simulink model "Simulation_DOA_rearanged"  (R2020b)
settings: Solver=ode4  StartTime=0.0  StopTime=timeToStop  FixedStep=1e-7  RelTol=1e-3
values from neighbouring files (symbols this model uses):
  f_range = [20e3 45e3]    [Init.m]
  FFT_LENGTH = 256    [Init.m]
  noise_on_off = false    [Init.m]
  noise_type = 1    [Init.m]
  Sampling_rate = 256e3    (= 256000)    [Init.m]
  timePerSample = 1/250e3    (= 4e-06)    [Init.m]
undefined symbols (not defined in the file or in its folder): Coeff_rect, InvMp, ProjectRate, RotX, runSim, SampleEstimate
libraries: dspsigops x25, dspsrcs4 x8, dsphdlmathfun x4, dsphdlxfrm x4, simulink x1, hdlsllib x1
(part 1 of 2)
settings Model: Creator=tigro  LastModifiedBy=franc
settings OptimizationCC: BlockReduction=off  ConditionallyExecuteInputs=off  DefaultParameterBehavior=Inlined  OptimizeBlockIOStorage=off  EnhancedBackFolding=on  PassReuseOutputArgsAs=Individual arguments  OptimizeBlockOrder=speed  DifferentSizesBufferReuse=on  EfficientTunableParamExpr=on
settings DebuggingCC: AlgebraicLoopMsg=error  ParameterOverflowMsg=none  ParameterTunabilityLossMsg=error
settings HardwareCC: ProdBitPerPointer=32  ProdBitPerSizeT=32  ProdBitPerPtrDiffT=32  ProdLargestAtomicFloat=None  ProdIntDivRoundTo=Undefined  ProdEndianess=Unspecified  ProdWordSize=32  ProdHWDeviceType=ASIC/FPGA->ASIC/FPGA  TargetBitPerPointer=64  TargetBitPerSizeT=64  TargetBitPerPtrDiffT=64  TargetLongLongMode=on  TargetIntDivRoundTo=Zero  TargetEndianess=LittleEndian  TargetWordSize=64  TargetHWDeviceType=Generic->Custom  ProdEqTarget=off
settings SFSimCC: MATLABDynamicMemAlloc=off
settings RTWCC: Description=SystemVerilog DPI Component Generator  SystemTargetFile=systemverilog_dpi_ert.tlc  TemplateMakefile=systemverilog_dpi_ert_default_tmf
settings CodeAppCC: ForceParamTrailComments=on  IgnoreCustomStorageClasses=off  MaxIdLength=256  OperatorAnnotations=on  SimulinkDataObjDesc=on  SFDataObjDesc=on  InsertBlockDesc=on
settings DPIERTTargetCC: TargetFcnLib=ansi_tfl_table_tmw.mat  GenFloatMathFcnCalls=NOT IN USE  TargetLangStandard=C89/C90 (ANSI)  CodeReplacementLibrary=None  UtilityFuncGeneration=Auto  MultiwordTypeDef=System defined  MultiwordLength=2048  DynamicStringBufferSize=256  GenerateFullHeader=on  InferredTypesCompatibility=off  GenerateSampleERTMain=off  GenerateTestInterfaces=off  ModelReferenceCompliant=on  ParMdlRefBuildCompliant=on  CompOptLevelCompliant=off  ConcurrentExecutionCompliant=off  IncludeMdlTerminateFcn=on  CombineOutputUpdateFcns=off  CombineSignalStateStructs=on  GroupInternalDataByFunction=off  SuppressErrorStatus=off  IncludeFileDelimiter=Auto  ERTCustomFileBanners=on  SupportAbsoluteTime=on  LogVarNameModifier=rt_  MatFileLogging=off  CodeInterfacePackaging=Reusable function  PurelyIntegerCode=off  SupportNonFinite=on  SupportComplex=on  SupportContinuousTime=on  SupportNonInlinedSFcns=on  RemoveDisableFunc=off  RemoveResetFunc=on  SupportVariableSizeSignals=off  ParenthesesLevel=Nominal  CastingMode=Nominal  MATLABClassNameForMDSCustomization=Simulink.SoftwareTarget.TargetSpecificTriggerConfigurationBase  ModelStepFunctionPrototypeControlCompliant=on  CPPClassGenCompliant=off  AutosarCompliant=off  MDXCompliant=off  GRTInterface=off  GenerateAllocFcn=on  UseToolchainInfoCompliant=on  GenerateSharedConstants=on  CoderGroups=[]  AccessMethods=[]  LookupTableObjectStructAxisOrder=1,2,3,4,...  LUTObjectStructOrderExplicitValues=Size,Breakpoints,Table  LUTObjectStructOrderEvenSpacing=Size,Breakpoints,Table  ArrayLayout=Column-major  UnsupportedSFcnMsg=error  ERTHeaderFileRootName=$R$E  ERTSourceFileRootName=$R$E  ERTDataFileRootName=$R_data  GenerateASAP2=off  DSAsUniqueAccess=off  ExtMode=off  ExtModeTransport=0  ExtModeStaticAlloc=off  ExtModeStaticAllocSize=1000000  ExtModeTesting=off  ExtModeMexFile=ext_comm  ExtModeIntrfLevel=Level1  InlinedParameterPlacement=NonHierarchical  TargetOS=BareBoardExample  MultiInstanceErrorCode=Error  RootIOFormat=Part of model data structure  RTWCAPISignals=on  RTWCAPIParams=off  RTWCAPIStates=off  RTWCAPIRootIO=off  ERTSrcFileBannerTemplate=ert_code_template.cgt  ERTHdrFileBannerTemplate=ert_code_template.cgt  ERTDataSrcFileTemplate=ert_code_template.cgt  ERTDataHdrFileTemplate=ert_code_template.cgt  ERTCustomFileTemplate=example_file_process.tlc  EnableDataOwnership=off  SignalDisplayLevel=10  ParamTuneLevel=10  GlobalDataDefinition=Auto  DataDefinitionFile=global.c  GlobalDataReference=Auto  ERTFilePackagingFormat=Modular  RateTransitionBlockCode=Inline  DataReferenceFile=global.h  PreserveExpressionOrder=off  PreserveIfCondition=off  ConvertIfToSwitch=on  PreserveExternInFcnDecls=on  PreserveStaticInFcnDecls=on  SuppressUnreachableDefaultCases=on  EnableSignedLeftShifts=on  EnableSignedRightShifts=on  IndentStyle=K&R  IndentSize=2  NewlineStyle=Default  MaxLineWidth=80  EnableUserReplacementTypes=off  MaxIdInt64=MAX_int64_T  MinIdInt64=MIN_int64_T  MaxIdUint64=MAX_uint64_T  MaxIdInt32=MAX_int32_T  MinIdInt32=MIN_int32_T  MaxIdUint32=MAX_uint32_T  MaxIdInt16=MAX_int16_T  MinIdInt16=MIN_int16_T  MaxIdUint16=MAX_uint16_T  MaxIdInt8=MAX_int8_T  MinIdInt8=MIN_int8_T  MaxIdUint8=MAX_uint8_T  BooleanTrueId=true  BooleanFalseId=false  MemSecPackage=--- None ---  MemSecDataConstants=Default  MemSecDataIO=Default  MemSecDataInternal=Default  MemSecDataParameters=Default  MemSecFuncInitTerm=Default  MemSecFuncExecute=Default  MemSecFuncSharedUtil=Default  GroupConstants=Default  GroupRootInputs=Default  GroupRootOutputs=Default  GroupInternal=Default  GroupParameters=Default  GroupDataTransfer=Default  GroupSharedLocalDataStores=Default  GroupInstanceSpecificParameters=Default  GroupModelData=Default  ArrayContainerType=C-style array  DPICustomizeSystemVerilogCode=off  DPISystemVerilogTemplate=svdpi_event.vgt  DPIReportRunTimeError=off  DPIRunTimeErrorSeverity=Fatal  DPIGenerateTestBench=off  DPITestBenchSimulator=Mentor Graphics Questasim  DPITestPointAccessFcnInterface=None  DPIFixedPointDataType=CompatibleCType  DPIPortConnection=Port list  DPICompositeDataType=Flattened

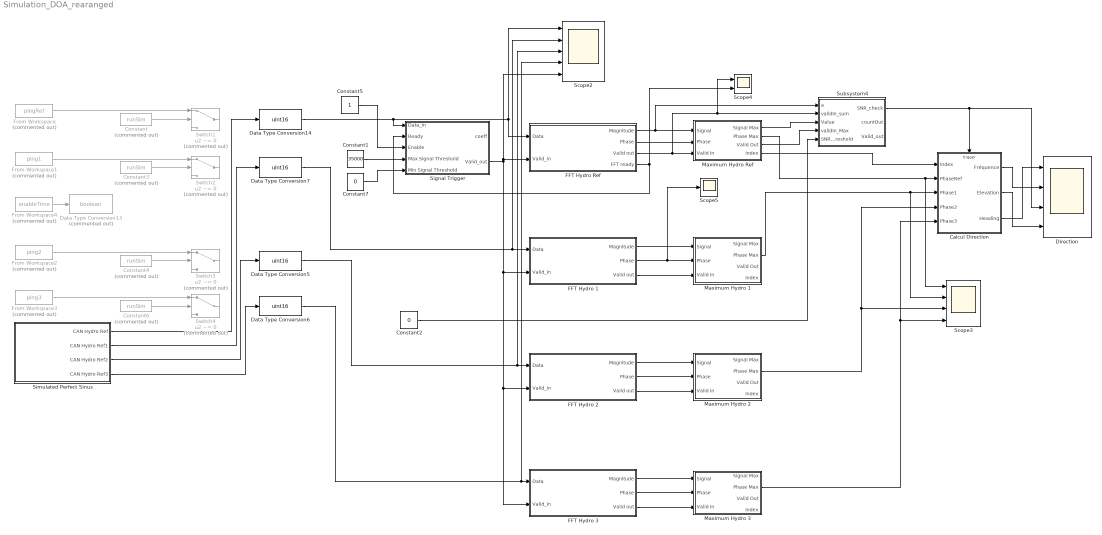
== system Simulation_DOA_rearanged ==
  Calcul Direction : Subsystem
  Constant{,3..4,6} (4 alike) : Constant  Commented=on  Value=runSim  SampleTime=-1
  Constant1 : Constant  Value=35000  OutDataTypeStr=uint16  SampleTime=-1
  Constant2 : Constant  Value=0  OutDataTypeStr=uint16  SampleTime=-1
  Constant5 : Constant  OutDataTypeStr=boolean
  Constant7 : Constant  Value=0  OutDataTypeStr=uint16  SampleTime=-1
  Data Type Conversion13 : DataTypeConversion  Commented=on  OutDataTypeStr=boolean
  Data Type Conversion{5..7,14} (4 alike) : DataTypeConversion  OutMax=[65535]  OutDataTypeStr=uint16
  Direction : Scope  NumInputPorts=4
  FFT Hydro 1 : Subsystem
  FFT Hydro 2 : Subsystem
  FFT Hydro 3 : Subsystem
  FFT Hydro Ref : Subsystem
  From Workspace : FromWorkspace  Commented=on  VariableName=pingRef  SampleTime=1/SampleEstimate  Interpolate=off  OutputAfterFinalValue=Setting to zero
  From Workspace1 : FromWorkspace  Commented=on  VariableName=ping1  SampleTime=1/SampleEstimate  Interpolate=off  OutputAfterFinalValue=Setting to zero
  From Workspace2 : FromWorkspace  Commented=on  VariableName=ping2  SampleTime=1/SampleEstimate  Interpolate=off  OutputAfterFinalValue=Setting to zero
  From Workspace3 : FromWorkspace  Commented=on  VariableName=ping3  SampleTime=1/SampleEstimate  Interpolate=off  OutputAfterFinalValue=Setting to zero
  From Workspace4 : FromWorkspace  Commented=on  VariableName=enableTime  SampleTime=1/ProjectRate  Interpolate=off  OutputAfterFinalValue=Setting to zero
  Maximum Hydro 1 : Subsystem
  Maximum Hydro 2 : Subsystem
  Maximum Hydro 3 : Subsystem
  Maximum Hydro Ref : Subsystem
  Scope2 : Scope  NumInputPorts=5
  Scope3 : Scope  NumInputPorts=4
  Scope4 : Scope  NumInputPorts=2
  Scope5 : Scope
  Signal Trigger : Subsystem
  Simulated Perfect Sinus : Subsystem
  Subsystem4 : Subsystem
  Switch{1..4} (4 alike) : Switch  Commented=on  Criteria=u2 ~= 0
  wires:
  Maximum Hydro Ref/1(Signal Max) -> Subsystem4/3(" Value")
  Data Type Conversion14/1 -> Signal Trigger/1(Data_in), Scope2/1, FFT Hydro Ref/1(Data)
  Data Type Conversion7/1 -> Scope2/2, FFT Hydro 1/1(Data)
  Data Type Conversion6/1 -> FFT Hydro 3/1(Data), Scope2/4
  FFT Hydro Ref/2(Phase) -> Maximum Hydro Ref/2(Phase)
  Maximum Hydro Ref/2(Phase Max) -> Scope3/1, Calcul Direction/2(PhaseRef)
  Maximum Hydro 1/2(Phase Max) -> Scope3/2, Calcul Direction/3(Phase1)
  Maximum Hydro 2/2(Phase Max) -> Calcul Direction/4(Phase2), Scope3/3
  Maximum Hydro 3/2(Phase Max) -> Calcul Direction/5(Phase3), Scope3/4
  Signal Trigger/2(Valid_out) -> Scope2/5, FFT Hydro Ref/2(Valid_in), FFT Hydro 3/2(Valid_in), FFT Hydro 2/2(Valid_in), FFT Hydro 1/2(Valid_in)
  FFT Hydro 1/1(Magnitude) -> Maximum Hydro 1/1(Signal)
  FFT Hydro 1/2(Phase) -> Scope5/1, Maximum Hydro 1/2(Phase)
  FFT Hydro 1/3(Valid out) -> Maximum Hydro 1/3(Valid In)
  FFT Hydro 2/1(Magnitude) -> Maximum Hydro 2/1(Signal)
  FFT Hydro 2/2(Phase) -> Maximum Hydro 2/2(Phase)
  FFT Hydro 2/3(Valid out) -> Maximum Hydro 2/3(Valid In)
  FFT Hydro 3/1(Magnitude) -> Maximum Hydro 3/1(Signal)
  FFT Hydro 3/2(Phase) -> Maximum Hydro 3/2(Phase)
  FFT Hydro 3/3(Valid out) -> Maximum Hydro 3/3(Valid In)
  Maximum Hydro Ref/3(Valid Out) -> Subsystem4/4(validIn_Max)
  FFT Hydro Ref/3(Valid out) -> Maximum Hydro Ref/3(Valid In), Scope4/1, Subsystem4/2(validIn_sum)
  Calcul Direction/1(Fréquence) -> Direction/2
  FFT Hydro Ref/1(Magnitude) -> Maximum Hydro Ref/1(Signal), Subsystem4/1(a)
  Subsystem4/1(SNR_check) -> Calcul Direction/Trigger, Direction/3
  Constant1/1 -> Signal Trigger/4(Max Signal Threshold)
  Constant2/1 -> Subsystem4/5(SNR_Threshold)
  Calcul Direction/2(Elevation) -> Direction/4
  From Workspace/1 -> Switch1/1
  From Workspace1/1 -> Switch2/1
  From Workspace2/1 -> Switch3/1
  From Workspace3/1 -> Switch4/1
  Constant/1 -> Switch1/2
  Constant3/1 -> Switch2/2
  Constant4/1 -> Switch3/2
  Constant6/1 -> Switch4/2
  FFT Hydro Ref/4(FFT ready) -> Scope4/2, Signal Trigger/2(Ready)
  From Workspace4/1 -> Data Type Conversion13/1
  Simulated Perfect Sinus/1(CAN Hydro Ref) -> Data Type Conversion14/1
  Simulated Perfect Sinus/2(CAN Hydro Ref1) -> Data Type Conversion7/1
  Simulated Perfect Sinus/3(CAN Hydro Ref2) -> Data Type Conversion5/1
  Simulated Perfect Sinus/4(CAN Hydro Ref3) -> Data Type Conversion6/1
  Constant7/1 -> Signal Trigger/5(Min Signal Threshold)
  Data Type Conversion5/1 -> Scope2/3, FFT Hydro 2/1(Data)
  Maximum Hydro Ref/4(Index) -> Calcul Direction/1(Index)
  Calcul Direction/3(Heading) -> Direction/1
  Constant5/1 -> Signal Trigger/3(Enable)

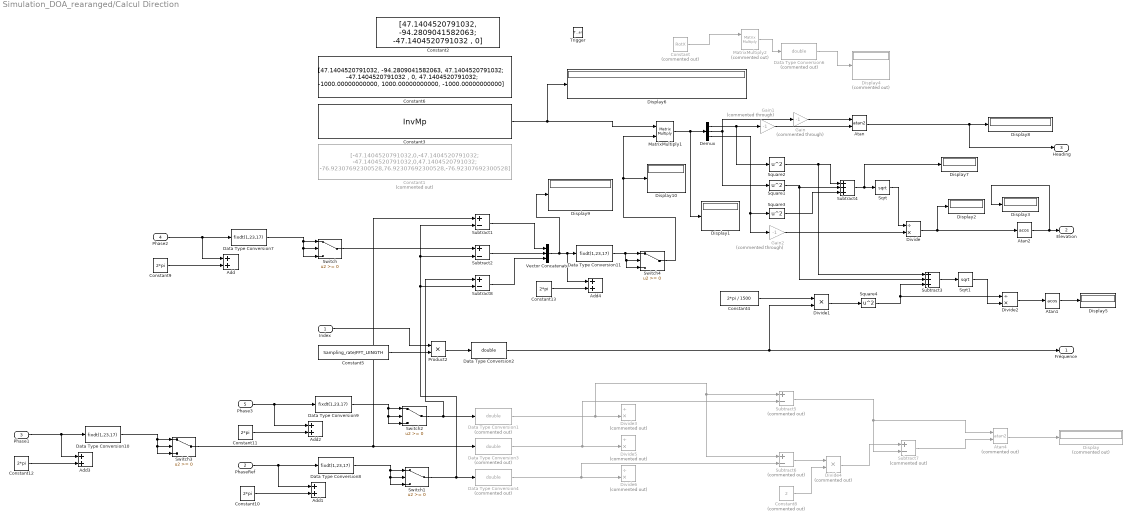
== system Simulation_DOA_rearanged/Calcul Direction ==
  Index : Inport
  PhaseRef : Inport  Port=2
  Phase1 : Inport  Port=3
  Phase2 : Inport  Port=4
  Phase3 : Inport  Port=5
  Trigger : TriggerPort  VariantControl=Variant  PortDimensions=1
  Add{,1..4} (5 alike) : Sum
  Atan : Trigonometry  Operator=atan2  ApproximationMethod=CORDIC  OutputSignalType=real
  Atan1 : Trigonometry  Operator=acos  ApproximationMethod=CORDIC  OutputSignalType=real
  Atan2 : Trigonometry  Operator=acos  ApproximationMethod=CORDIC  OutputSignalType=real
  Atan4 : Trigonometry  Commented=on  Operator=atan2  ApproximationMethod=CORDIC  OutputSignalType=real
  Constant : Constant  Commented=on  Value=RotX
  Constant1 : Constant  Commented=on  Value=|  VectorParams1D=off  OutDataTypeStr=fixdt(1,15,7)
      | [-47.1404520791032,0,-47.1404520791032; -47.1404520791032,0,47.1404520791032;
      | -76.92307692300528,76.92307692300528,-76.92307692300528]
  Constant{9..13} (5 alike) : Constant  Value=2*pi  OutDataTypeStr=fixdt(0,16,12)  SampleTime=-1
  Constant2 : Constant  Value=|  VectorParams1D=off  OutDataTypeStr=fixdt(1,15,7)
      | [47.1404520791032,    -94.2809041582063;
      | -47.1404520791032 ,   0]
  Constant3 : Constant  Value=InvMp  VectorParams1D=off  OutDataTypeStr=fixdt(1,32,16)
  Constant4 : Constant  Value=2*pi / 1500
  Constant5 : Constant  Value=Sampling_rate/FFT_LENGTH  OutDataTypeStr=Inherit: Inherit via back propagation  SampleTime=-1
  Constant6 : Constant  Value=|  VectorParams1D=off  OutDataTypeStr=fixdt(1,15,7)
      | [47.1404520791032,    -94.2809041582063,    47.1404520791032;
      | -47.1404520791032 ,   0,    47.1404520791032;
      | -1000.00000000000,   1000.00000000000,    -1000.00000000000]
  Constant8 : Constant  Commented=on  Value=2  OutDataTypeStr=uint8
  Data Type Conversion{1,3..4,6} (4 alike) : DataTypeConversion  Commented=on  OutDataTypeStr=double
  Data Type Conversion{7..11} (5 alike) : DataTypeConversion  OutDataTypeStr=fixdt(1,23,17)
  Data Type Conversion2 : DataTypeConversion  OutDataTypeStr=double
  Demux : Demux  Outputs=3
  Display : Display  Commented=on
      settings: Decimation=8
  Display{1..3,5..10} (9 alike) : Display
      Display8 settings: Decimation=8
  Display4 : Display  Commented=on
  Divide : Product  Inputs=/*
  Divide1 : Product  Inputs=**  RndMeth=Zero  SaturateOnIntegerOverflow=on
  Divide2 : Product  Inputs=/*
  Divide3 : Product  Commented=on  Inputs=/*  RndMeth=Zero  SaturateOnIntegerOverflow=on
  Divide4 : Product  Commented=on  Inputs=**  RndMeth=Zero  SaturateOnIntegerOverflow=on
  Divide5 : Product  Commented=on  Inputs=/*  RndMeth=Zero  SaturateOnIntegerOverflow=on
  Divide6 : Product  Commented=on  Inputs=/*  RndMeth=Zero  SaturateOnIntegerOverflow=on
  Gain : Gain  Commented=through  Gain=-1
  Gain1 : Gain  Commented=through  Gain=-1
  Gain2 : Gain  Commented=through  Gain=-1
  MatrixMultiply1 : Product  Multiplication=Matrix(*)
  MatrixMultiply2 : Product  Commented=on  Multiplication=Matrix(*)
  Product2 : Product
  Sqrt : Sqrt  OutDataTypeStr=double  SaturateOnIntegerOverflow=on
  Sqrt1 : Sqrt  OutDataTypeStr=double  SaturateOnIntegerOverflow=on
  Square{1..4} (4 alike) : Math  Operator=square  SignedPower=on  RndMeth=Zero  SaturateOnIntegerOverflow=on  OutDataTypeStr=Inherit: Inherit via internal rule
  Subtract1 : Sum  Inputs=+-
  Subtract2 : Sum  Inputs=+-
  Subtract3 : Sum  Inputs=+++
  Subtract4 : Sum  Inputs=+++
  Subtract5 : Sum  Commented=on  Inputs=+-
  Subtract6 : Sum  Commented=on  Inputs=+-
  Subtract7 : Sum  Commented=on  Inputs=+-
  Subtract8 : Sum  Inputs=+-
  Switch{,1..4} (5 alike) : Switch
  Vector Concatenate : Concatenate  NumInputs=3  Mode=Multidimensional array
  Fréquence : Outport  InitialOutput=0
  Elevation : Outport  Port=2  InitialOutput=0
  Heading : Outport  Port=3  InitialOutput=0
  wires:
  Constant5/1 -> Product2/2
  Square2/1 -> Subtract3/1, Subtract4/1
  Demux/1 -> Square2/1, Gain1/1
  Product2/1 -> Data Type Conversion2/1
  Subtract4/1 -> Display7/1, Sqrt/1
  Index/1 -> Product2/1
  Square1/1 -> Subtract3/2, Subtract4/2
  Square3/1 -> Subtract4/3
  Sqrt/1 -> Divide/1
  Atan2/1 -> Display3/1, Elevation/1
  Demux/2 -> Gain/1, Square1/1
  MatrixMultiply1/1 -> Display1/1, Demux/1
  Demux/3 -> Gain2/1, Square3/1
  Constant3/1 -> Display6/1, MatrixMultiply1/1
  Constant/1 -> MatrixMultiply2/1
  MatrixMultiply2/1 -> Data Type Conversion6/1
  Data Type Conversion6/1 -> Display4/1
  Constant4/1 -> Divide1/1
  Divide1/1 -> Square4/1
  Subtract3/1 -> Sqrt1/1
  Square4/1 -> Divide2/1, Subtract3/3
  Sqrt1/1 -> Divide2/2
  Divide2/1 -> Atan1/1
  Atan1/1 -> Display5/1
  Vector Concatenate/1 -> Display9/1, Add4/1, Data Type Conversion11/1
  Divide4/1 -> Subtract7/1
  Subtract7/1 -> Atan4/2
  Subtract6/1 -> Divide4/1
  Constant8/1 -> Divide4/2
  Subtract5/1 -> Atan4/1, Subtract7/2
  Atan4/1 -> Display/1
  Data Type Conversion1/1 -> Divide3/2, Subtract6/1, Subtract5/1
  Data Type Conversion3/1 -> Divide5/2, Subtract5/2
  Data Type Conversion4/1 -> Divide6/2, Subtract6/2
  Data Type Conversion2/1 -> Divide1/2, Fréquence/1
  Atan/1 -> Heading/1, Display8/1
  Switch/1 -> Subtract2/1
  Constant9/1 -> Add/2
  Phase2/1 -> Add/1, Data Type Conversion7/1
  Data Type Conversion7/1 -> Switch/3, Switch/2, Switch/1
  Constant10/1 -> Add1/2
  Data Type Conversion8/1 -> Switch1/3, Switch1/2, Switch1/1
  Constant11/1 -> Add2/2
  Data Type Conversion9/1 -> Switch2/3, Switch2/2, Switch2/1
  Constant12/1 -> Add3/2
  Data Type Conversion10/1 -> Switch3/3, Switch3/2, Switch3/1
  Switch1/1 -> Subtract8/2, Subtract2/2, Subtract1/2, Data Type Conversion4/1
  PhaseRef/1 -> Add1/1, Data Type Conversion8/1
  Switch2/1 -> Subtract8/1, Data Type Conversion1/1
  Phase3/1 -> Add2/1, Data Type Conversion9/1
  Switch3/1 -> Data Type Conversion3/1, Subtract1/1
  Phase1/1 -> Add3/1, Data Type Conversion10/1
  Data Type Conversion11/1 -> Switch4/3, Switch4/2, Switch4/1
  Constant13/1 -> Add4/2
  Switch4/1 -> Display10/1, MatrixMultiply1/2
  Subtract1/1 -> Vector Concatenate/1
  Subtract2/1 -> Vector Concatenate/2
  Subtract8/1 -> Vector Concatenate/3
  Gain/1 -> Atan/1
  Gain1/1 -> Atan/2
  Divide/1 -> Atan2/1, Display2/1
  Gain2/1 -> Divide/2

== system Simulation_DOA_rearanged/FFT Hydro 1 ==
  Data : Inport
  Valid_in : Inport  Port=2
  Complex to Magnitude-Angle HDL Optimized : dsphdlmathfun/Complex to Magnitude-Angle HDL Optimized  NumIterationsSource=Property  NumIterations=CORDIC_Estimation  OutputFormat=Magnitude and angle  AngleFormat=Radians  ScaleOutput=on  SimulateUsing=Code generation
      settings: SourceProductBaseCode=DS
  FFT HDL Optimized : dsphdlxfrm/FFT HDL Optimized  FFTLength=FFT_LENGTH  Architecture=Burst Radix 2  ComplexMultiplication=Use 3 multipliers and 5 adders  BitReversedOutput=off  BitReversedInput=off  Normalize=on  SimulateUsing=Code generation  RoundingMethod=Floor  ResetInputPort=off  StartOutputPort=off  EndOutputPort=on
      settings: SourceProductBaseCode=DS
  Magnitude : Outport
  Phase : Outport  Port=2
  Valid out : Outport  Port=3
  wires:
  Valid_in/1 -> FFT HDL Optimized/2
  FFT HDL Optimized/1 -> Complex to Magnitude-Angle HDL Optimized/1
  Complex to Magnitude-Angle HDL Optimized/1 -> Magnitude/1
  Complex to Magnitude-Angle HDL Optimized/2 -> Phase/1
  Data/1 -> FFT HDL Optimized/1
  FFT HDL Optimized/3 -> Complex to Magnitude-Angle HDL Optimized/2
  Complex to Magnitude-Angle HDL Optimized/3 -> Valid out/1

== system Simulation_DOA_rearanged/FFT Hydro 2 ==
  Data : Inport
  Valid_in : Inport  Port=2
  Complex to Magnitude-Angle HDL Optimized : dsphdlmathfun/Complex to Magnitude-Angle HDL Optimized  NumIterationsSource=Property  NumIterations=CORDIC_Estimation  OutputFormat=Magnitude and angle  AngleFormat=Radians  ScaleOutput=on  SimulateUsing=Code generation
      settings: SourceProductBaseCode=DS
  FFT HDL Optimized : dsphdlxfrm/FFT HDL Optimized  FFTLength=FFT_LENGTH  Architecture=Burst Radix 2  ComplexMultiplication=Use 3 multipliers and 5 adders  BitReversedOutput=off  BitReversedInput=off  Normalize=on  SimulateUsing=Code generation  RoundingMethod=Floor  ResetInputPort=off  StartOutputPort=off  EndOutputPort=on
      settings: SourceProductBaseCode=DS
  Magnitude : Outport
  Phase : Outport  Port=2
  Valid out : Outport  Port=3
  wires:
  Valid_in/1 -> FFT HDL Optimized/2
  FFT HDL Optimized/1 -> Complex to Magnitude-Angle HDL Optimized/1
  Complex to Magnitude-Angle HDL Optimized/1 -> Magnitude/1
  Complex to Magnitude-Angle HDL Optimized/2 -> Phase/1
  Data/1 -> FFT HDL Optimized/1
  FFT HDL Optimized/3 -> Complex to Magnitude-Angle HDL Optimized/2
  Complex to Magnitude-Angle HDL Optimized/3 -> Valid out/1

== system Simulation_DOA_rearanged/FFT Hydro 3 ==
  Data : Inport
  Valid_in : Inport  Port=2
  Complex to Magnitude-Angle HDL Optimized : dsphdlmathfun/Complex to Magnitude-Angle HDL Optimized  NumIterationsSource=Property  NumIterations=CORDIC_Estimation  OutputFormat=Magnitude and angle  AngleFormat=Radians  ScaleOutput=on  SimulateUsing=Code generation
      settings: SourceProductBaseCode=DS
  FFT HDL Optimized : dsphdlxfrm/FFT HDL Optimized  FFTLength=FFT_LENGTH  Architecture=Burst Radix 2  ComplexMultiplication=Use 3 multipliers and 5 adders  BitReversedOutput=off  BitReversedInput=off  Normalize=on  SimulateUsing=Code generation  RoundingMethod=Floor  ResetInputPort=off  StartOutputPort=off  EndOutputPort=on
      settings: SourceProductBaseCode=DS
  Magnitude : Outport
  Phase : Outport  Port=2
  Valid out : Outport  Port=3
  wires:
  Valid_in/1 -> FFT HDL Optimized/2
  FFT HDL Optimized/1 -> Complex to Magnitude-Angle HDL Optimized/1
  Complex to Magnitude-Angle HDL Optimized/1 -> Magnitude/1
  Complex to Magnitude-Angle HDL Optimized/2 -> Phase/1
  Data/1 -> FFT HDL Optimized/1
  FFT HDL Optimized/3 -> Complex to Magnitude-Angle HDL Optimized/2
  Complex to Magnitude-Angle HDL Optimized/3 -> Valid out/1

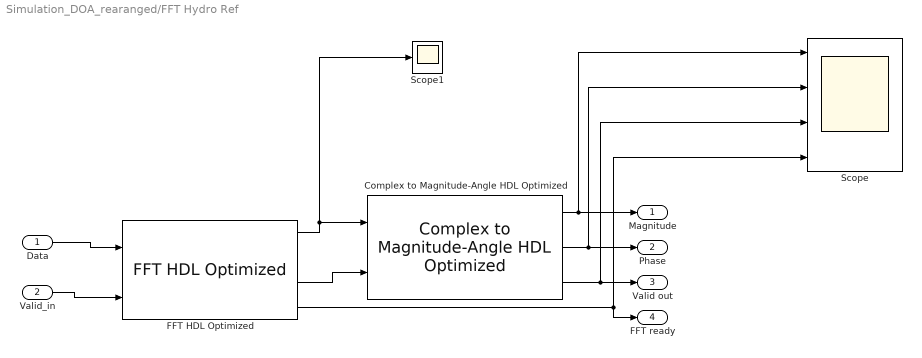
== system Simulation_DOA_rearanged/FFT Hydro Ref ==
  Data : Inport
  Valid_in : Inport  Port=2
  Complex to Magnitude-Angle HDL Optimized : dsphdlmathfun/Complex to Magnitude-Angle HDL Optimized  NumIterationsSource=Property  NumIterations=CORDIC_Estimation  OutputFormat=Magnitude and angle  AngleFormat=Radians  ScaleOutput=on  SimulateUsing=Code generation
      settings: SourceProductBaseCode=DS
  FFT HDL Optimized : dsphdlxfrm/FFT HDL Optimized  FFTLength=FFT_LENGTH  Architecture=Burst Radix 2  ComplexMultiplication=Use 3 multipliers and 5 adders  BitReversedOutput=off  BitReversedInput=off  Normalize=on  SimulateUsing=Code generation  RoundingMethod=Floor  ResetInputPort=off  StartOutputPort=off  EndOutputPort=on
      settings: SourceProductBaseCode=DS
  Scope : Scope  NumInputPorts=4
  Scope1 : Scope
  Magnitude : Outport
  Phase : Outport  Port=2
  Valid out : Outport  Port=3
  FFT ready : Outport  Port=4
  wires:
  Valid_in/1 -> FFT HDL Optimized/2
  FFT HDL Optimized/1 -> Complex to Magnitude-Angle HDL Optimized/1, Scope1/1
  Complex to Magnitude-Angle HDL Optimized/1 -> Scope/1, Magnitude/1
  Complex to Magnitude-Angle HDL Optimized/2 -> Scope/2, Phase/1
  Data/1 -> FFT HDL Optimized/1
  FFT HDL Optimized/3 -> Complex to Magnitude-Angle HDL Optimized/2
  Complex to Magnitude-Angle HDL Optimized/3 -> Scope/3, Valid out/1
  FFT HDL Optimized/4 -> FFT ready/1, Scope/4

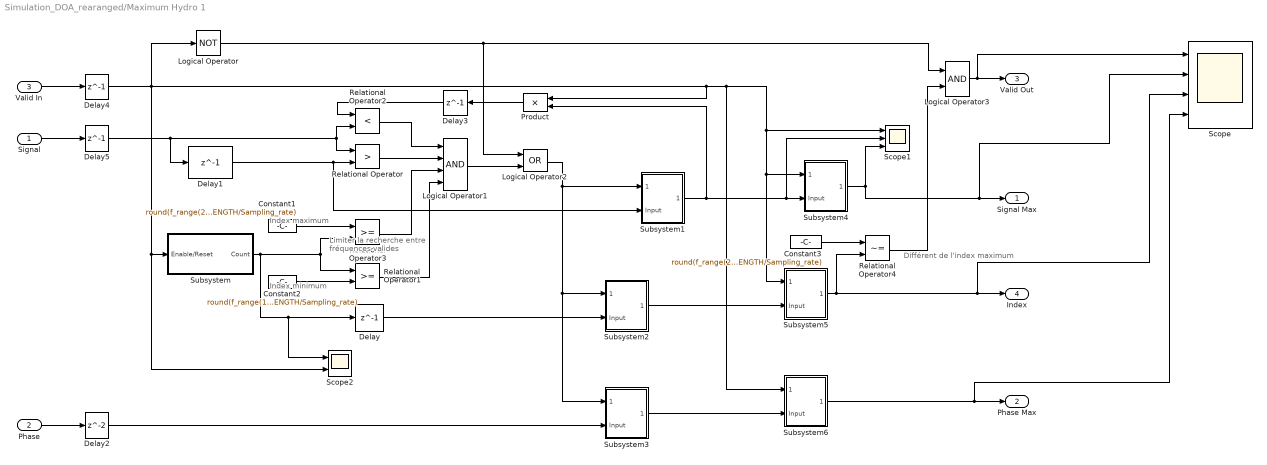
== system Simulation_DOA_rearanged/Maximum Hydro 1 ==
  note: Index minimum
  note: Index maximum
  note: Limiter la recherche
      | entre fréquences valides
  note: Différent de l'index
      | maximum
  Signal : Inport
  Phase : Inport  Port=2
  Valid In : Inport  Port=3
  Constant1 : Constant  Value=round(f_range(2)*FFT_LENGTH/Sampling_rate)  OutDataTypeStr=fixdt(0,6)  SampleTime=-1
  Constant2 : Constant  Value=round(f_range(1)*FFT_LENGTH/Sampling_rate)  OutDataTypeStr=fixdt(0,6)  SampleTime=-1
  Constant3 : Constant  Value=round(f_range(2)*FFT_LENGTH/Sampling_rate)  OutDataTypeStr=fixdt(0,6)  SampleTime=-1
  Delay : Delay  DelayLength=1  InitialCondition=0
  Delay{1,3..5} (4 alike) : Delay  DelayLength=1  InitialCondition=0  UseCircularBuffer=on
  Delay2 : Delay  InitialCondition=0  UseCircularBuffer=on
  Logical Operator : Logic  Operator=NOT  IconShape=distinctive  AllPortsSameDT=off  OutDataTypeStr=boolean
  Logical Operator1 : Logic  Inputs=4  AllPortsSameDT=off  OutDataTypeStr=boolean
  Logical Operator2 : Logic  Operator=OR  AllPortsSameDT=off  OutDataTypeStr=boolean
  Logical Operator3 : Logic  AllPortsSameDT=off  OutDataTypeStr=boolean
  Product : Product
  Relational Operator : RelationalOperator  Operator=>  OutDataTypeStr=boolean  RndMeth=Nearest
  Relational Operator1 : RelationalOperator  OutDataTypeStr=boolean  RndMeth=Nearest
  Relational Operator2 : RelationalOperator  Operator=<  OutDataTypeStr=boolean  RndMeth=Nearest
  Relational Operator3 : RelationalOperator  OutDataTypeStr=boolean  RndMeth=Nearest
  Relational Operator4 : RelationalOperator  Operator=~=  OutDataTypeStr=boolean  RndMeth=Nearest
  Scope : Scope  NumInputPorts=4
  Scope1 : Scope  NumInputPorts=3
  Scope2 : Scope  NumInputPorts=2
  Subsystem : Subsystem
  Subsystem1 : Subsystem  TreatAsAtomicUnit=on
  Subsystem2 : Subsystem  TreatAsAtomicUnit=on
  Subsystem3 : Subsystem  TreatAsAtomicUnit=on
  Subsystem4 : Subsystem  TreatAsAtomicUnit=on
  Subsystem5 : Subsystem  TreatAsAtomicUnit=on
  Subsystem6 : Subsystem  TreatAsAtomicUnit=on
  Signal Max : Outport  VectorParamsAs1DForOutWhenUnconnected=off
  Phase Max : Outport  Port=2  VectorParamsAs1DForOutWhenUnconnected=off
  Valid Out : Outport  Port=3  VectorParamsAs1DForOutWhenUnconnected=off
  Index : Outport  Port=4  VectorParamsAs1DForOutWhenUnconnected=off
  wires:
  Subsystem1/1(" ") -> Product/2, Subsystem4/2(Input), Scope1/2
  Signal/1 -> Delay5/1
  Subsystem2/1(" ") -> Subsystem5/2(Input)
  Valid In/1 -> Delay4/1
  Delay1/1 -> Subsystem1/2(Input), Relational Operator/2
  Subsystem4/1(" ") -> Scope/2, Signal Max/1, Scope1/3
  Constant2/1 -> Relational Operator1/2
  Subsystem3/1(" ") -> Subsystem6/2(Input)
  Phase/1 -> Delay2/1
  Subsystem6/1(" ") -> Phase Max/1, Scope/4
  Subsystem/1(Count) -> Scope2/1, Delay/1, Relational Operator1/1, Relational Operator3/2
  Relational Operator2/1 -> Logical Operator1/1
  Relational Operator/1 -> Logical Operator1/2
  Delay3/1 -> Relational Operator2/1
  Product/1 -> Delay3/1
  Delay4/1 -> Logical Operator/1, Subsystem6/1(Trigger), Subsystem5/1(Trigger), Subsystem4/1(Trigger), Scope1/1, Product/1, Scope2/2, Subsystem/1(Enable/Reset)
  Delay5/1 -> Relational Operator2/2, Relational Operator/1, Delay1/1
  Delay2/1 -> Subsystem3/2(Input)
  Constant1/1 -> Relational Operator3/1
  Relational Operator1/1 -> Logical Operator1/4
  Logical Operator/1 -> Logical Operator2/1, Logical Operator3/1
  Logical Operator3/1 -> Scope/1, Valid Out/1
  Relational Operator3/1 -> Logical Operator1/3
  Relational Operator4/1 -> Logical Operator3/2
  Constant3/1 -> Relational Operator4/1
  Logical Operator1/1 -> Logical Operator2/2
  Logical Operator2/1 -> Subsystem1/1(Trigger), Subsystem3/1(Trigger), Subsystem2/1(Trigger)
  Delay/1 -> Subsystem2/2(Input)
  Subsystem5/1(" ") -> Index/1, Scope/3, Relational Operator4/2

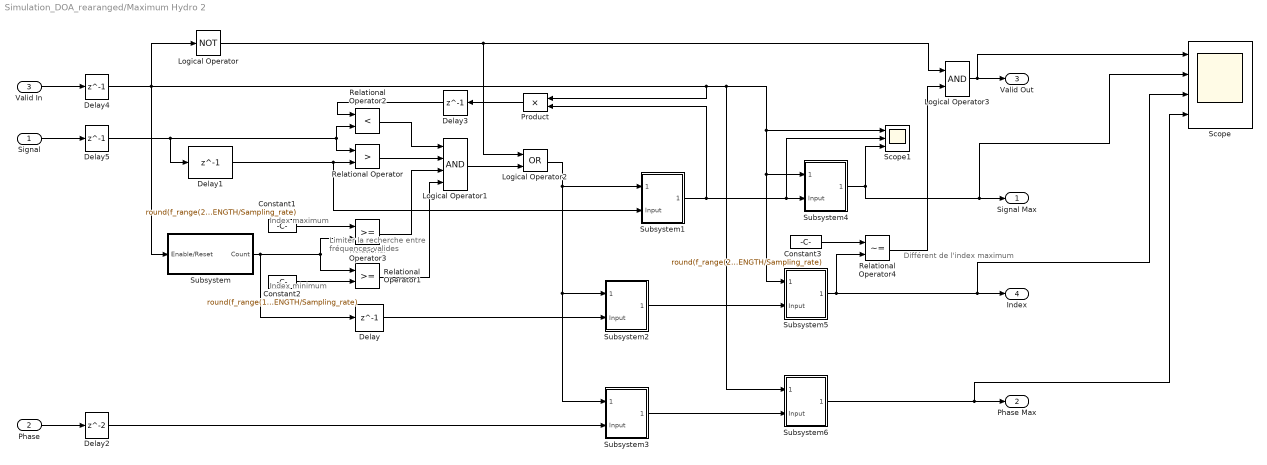
== system Simulation_DOA_rearanged/Maximum Hydro 2 ==
  note: Index minimum
  note: Index maximum
  note: Limiter la recherche
      | entre fréquences valides
  note: Différent de l'index
      | maximum
  Signal : Inport
  Phase : Inport  Port=2
  Valid In : Inport  Port=3
  Constant1 : Constant  Value=round(f_range(2)*FFT_LENGTH/Sampling_rate)  OutDataTypeStr=fixdt(0,6)  SampleTime=-1
  Constant2 : Constant  Value=round(f_range(1)*FFT_LENGTH/Sampling_rate)  OutDataTypeStr=fixdt(0,6)  SampleTime=-1
  Constant3 : Constant  Value=round(f_range(2)*FFT_LENGTH/Sampling_rate)  OutDataTypeStr=fixdt(0,6)  SampleTime=-1
  Delay : Delay  DelayLength=1  InitialCondition=0
  Delay{1,3..5} (4 alike) : Delay  DelayLength=1  InitialCondition=0  UseCircularBuffer=on
  Delay2 : Delay  InitialCondition=0  UseCircularBuffer=on
  Logical Operator : Logic  Operator=NOT  IconShape=distinctive  AllPortsSameDT=off  OutDataTypeStr=boolean
  Logical Operator1 : Logic  Inputs=4  AllPortsSameDT=off  OutDataTypeStr=boolean
  Logical Operator2 : Logic  Operator=OR  AllPortsSameDT=off  OutDataTypeStr=boolean
  Logical Operator3 : Logic  AllPortsSameDT=off  OutDataTypeStr=boolean
  Product : Product
  Relational Operator : RelationalOperator  Operator=>  OutDataTypeStr=boolean  RndMeth=Nearest
  Relational Operator1 : RelationalOperator  OutDataTypeStr=boolean  RndMeth=Nearest
  Relational Operator2 : RelationalOperator  Operator=<  OutDataTypeStr=boolean  RndMeth=Nearest
  Relational Operator3 : RelationalOperator  OutDataTypeStr=boolean  RndMeth=Nearest
  Relational Operator4 : RelationalOperator  Operator=~=  OutDataTypeStr=boolean  RndMeth=Nearest
  Scope : Scope  NumInputPorts=4
  Scope1 : Scope  NumInputPorts=3
  Subsystem : Subsystem
  Subsystem1 : Subsystem  TreatAsAtomicUnit=on
  Subsystem2 : Subsystem  TreatAsAtomicUnit=on
  Subsystem3 : Subsystem  TreatAsAtomicUnit=on
  Subsystem4 : Subsystem  TreatAsAtomicUnit=on
  Subsystem5 : Subsystem  TreatAsAtomicUnit=on
  Subsystem6 : Subsystem  TreatAsAtomicUnit=on
  Signal Max : Outport  VectorParamsAs1DForOutWhenUnconnected=off
  Phase Max : Outport  Port=2  VectorParamsAs1DForOutWhenUnconnected=off
  Valid Out : Outport  Port=3  VectorParamsAs1DForOutWhenUnconnected=off
  Index : Outport  Port=4  VectorParamsAs1DForOutWhenUnconnected=off
  wires:
  Subsystem1/1(" ") -> Product/2, Subsystem4/2(Input), Scope1/2
  Signal/1 -> Delay5/1
  Subsystem2/1(" ") -> Subsystem5/2(Input)
  Valid In/1 -> Delay4/1
  Delay1/1 -> Subsystem1/2(Input), Relational Operator/2
  Subsystem4/1(" ") -> Scope/2, Signal Max/1, Scope1/3
  Constant2/1 -> Relational Operator1/2
  Subsystem3/1(" ") -> Subsystem6/2(Input)
  Phase/1 -> Delay2/1
  Subsystem6/1(" ") -> Phase Max/1, Scope/4
  Subsystem/1(Count) -> Delay/1, Relational Operator1/1, Relational Operator3/2
  Relational Operator2/1 -> Logical Operator1/1
  Relational Operator/1 -> Logical Operator1/2
  Delay3/1 -> Relational Operator2/1
  Product/1 -> Delay3/1
  Delay4/1 -> Logical Operator/1, Subsystem6/1(Trigger), Subsystem5/1(Trigger), Subsystem4/1(Trigger), Scope1/1, Product/1, Subsystem/1(Enable/Reset)
  Delay5/1 -> Relational Operator2/2, Relational Operator/1, Delay1/1
  Delay2/1 -> Subsystem3/2(Input)
  Constant1/1 -> Relational Operator3/1
  Relational Operator1/1 -> Logical Operator1/4
  Logical Operator/1 -> Logical Operator2/1, Logical Operator3/1
  Logical Operator3/1 -> Scope/1, Valid Out/1
  Relational Operator3/1 -> Logical Operator1/3
  Relational Operator4/1 -> Logical Operator3/2
  Constant3/1 -> Relational Operator4/1
  Logical Operator1/1 -> Logical Operator2/2
  Logical Operator2/1 -> Subsystem1/1(Trigger), Subsystem3/1(Trigger), Subsystem2/1(Trigger)
  Delay/1 -> Subsystem2/2(Input)
  Subsystem5/1(" ") -> Index/1, Scope/3, Relational Operator4/2

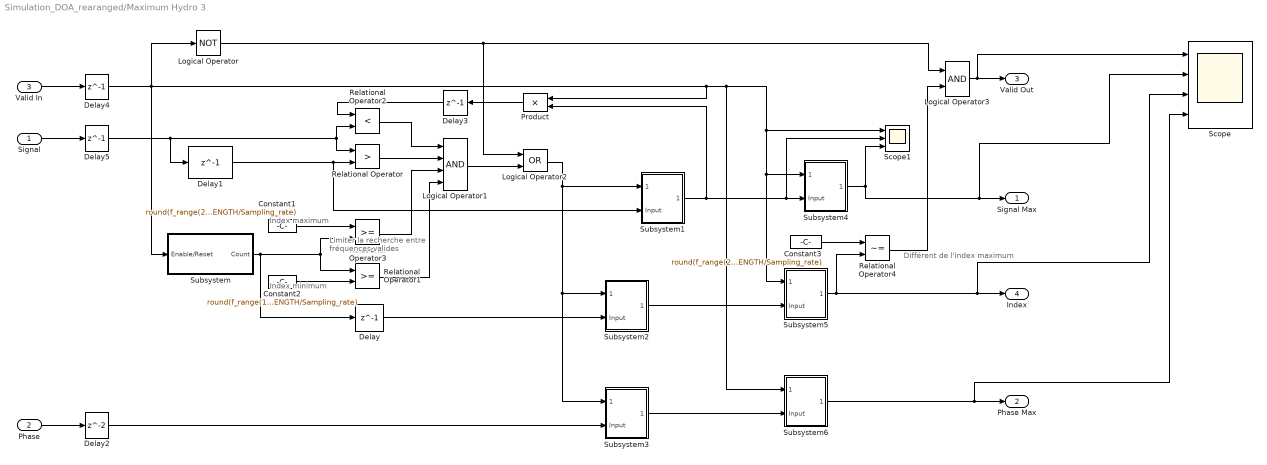
== system Simulation_DOA_rearanged/Maximum Hydro 3 ==
  note: Index minimum
  note: Index maximum
  note: Limiter la recherche
      | entre fréquences valides
  note: Différent de l'index
      | maximum
  Signal : Inport
  Phase : Inport  Port=2
  Valid In : Inport  Port=3
  Constant1 : Constant  Value=round(f_range(2)*FFT_LENGTH/Sampling_rate)  OutDataTypeStr=fixdt(0,6)  SampleTime=-1
  Constant2 : Constant  Value=round(f_range(1)*FFT_LENGTH/Sampling_rate)  OutDataTypeStr=fixdt(0,6)  SampleTime=-1
  Constant3 : Constant  Value=round(f_range(2)*FFT_LENGTH/Sampling_rate)  OutDataTypeStr=fixdt(0,6)  SampleTime=-1
  Delay : Delay  DelayLength=1  InitialCondition=0
  Delay{1,3..5} (4 alike) : Delay  DelayLength=1  InitialCondition=0  UseCircularBuffer=on
  Delay2 : Delay  InitialCondition=0  UseCircularBuffer=on
  Logical Operator : Logic  Operator=NOT  IconShape=distinctive  AllPortsSameDT=off  OutDataTypeStr=boolean
  Logical Operator1 : Logic  Inputs=4  AllPortsSameDT=off  OutDataTypeStr=boolean
  Logical Operator2 : Logic  Operator=OR  AllPortsSameDT=off  OutDataTypeStr=boolean
  Logical Operator3 : Logic  AllPortsSameDT=off  OutDataTypeStr=boolean
  Product : Product
  Relational Operator : RelationalOperator  Operator=>  OutDataTypeStr=boolean  RndMeth=Nearest
  Relational Operator1 : RelationalOperator  OutDataTypeStr=boolean  RndMeth=Nearest
  Relational Operator2 : RelationalOperator  Operator=<  OutDataTypeStr=boolean  RndMeth=Nearest
  Relational Operator3 : RelationalOperator  OutDataTypeStr=boolean  RndMeth=Nearest
  Relational Operator4 : RelationalOperator  Operator=~=  OutDataTypeStr=boolean  RndMeth=Nearest
  Scope : Scope  NumInputPorts=4
  Scope1 : Scope  NumInputPorts=3
  Subsystem : Subsystem
  Subsystem1 : Subsystem  TreatAsAtomicUnit=on
  Subsystem2 : Subsystem  TreatAsAtomicUnit=on
  Subsystem3 : Subsystem  TreatAsAtomicUnit=on
  Subsystem4 : Subsystem  TreatAsAtomicUnit=on
  Subsystem5 : Subsystem  TreatAsAtomicUnit=on
  Subsystem6 : Subsystem  TreatAsAtomicUnit=on
  Signal Max : Outport  VectorParamsAs1DForOutWhenUnconnected=off
  Phase Max : Outport  Port=2  VectorParamsAs1DForOutWhenUnconnected=off
  Valid Out : Outport  Port=3  VectorParamsAs1DForOutWhenUnconnected=off
  Index : Outport  Port=4  VectorParamsAs1DForOutWhenUnconnected=off
  wires:
  Subsystem1/1(" ") -> Product/2, Subsystem4/2(Input), Scope1/2
  Signal/1 -> Delay5/1
  Subsystem2/1(" ") -> Subsystem5/2(Input)
  Valid In/1 -> Delay4/1
  Delay1/1 -> Subsystem1/2(Input), Relational Operator/2
  Subsystem4/1(" ") -> Scope/2, Signal Max/1, Scope1/3
  Constant2/1 -> Relational Operator1/2
  Subsystem3/1(" ") -> Subsystem6/2(Input)
  Phase/1 -> Delay2/1
  Subsystem6/1(" ") -> Phase Max/1, Scope/4
  Subsystem/1(Count) -> Delay/1, Relational Operator1/1, Relational Operator3/2
  Relational Operator2/1 -> Logical Operator1/1
  Relational Operator/1 -> Logical Operator1/2
  Delay3/1 -> Relational Operator2/1
  Product/1 -> Delay3/1
  Delay4/1 -> Logical Operator/1, Subsystem6/1(Trigger), Subsystem5/1(Trigger), Subsystem4/1(Trigger), Scope1/1, Product/1, Subsystem/1(Enable/Reset)
  Delay5/1 -> Relational Operator2/2, Relational Operator/1, Delay1/1
  Delay2/1 -> Subsystem3/2(Input)
  Constant1/1 -> Relational Operator3/1
  Relational Operator1/1 -> Logical Operator1/4
  Logical Operator/1 -> Logical Operator2/1, Logical Operator3/1
  Logical Operator3/1 -> Scope/1, Valid Out/1
  Relational Operator3/1 -> Logical Operator1/3
  Relational Operator4/1 -> Logical Operator3/2
  Constant3/1 -> Relational Operator4/1
  Logical Operator1/1 -> Logical Operator2/2
  Logical Operator2/1 -> Subsystem1/1(Trigger), Subsystem3/1(Trigger), Subsystem2/1(Trigger)
  Delay/1 -> Subsystem2/2(Input)
  Subsystem5/1(" ") -> Index/1, Scope/3, Relational Operator4/2

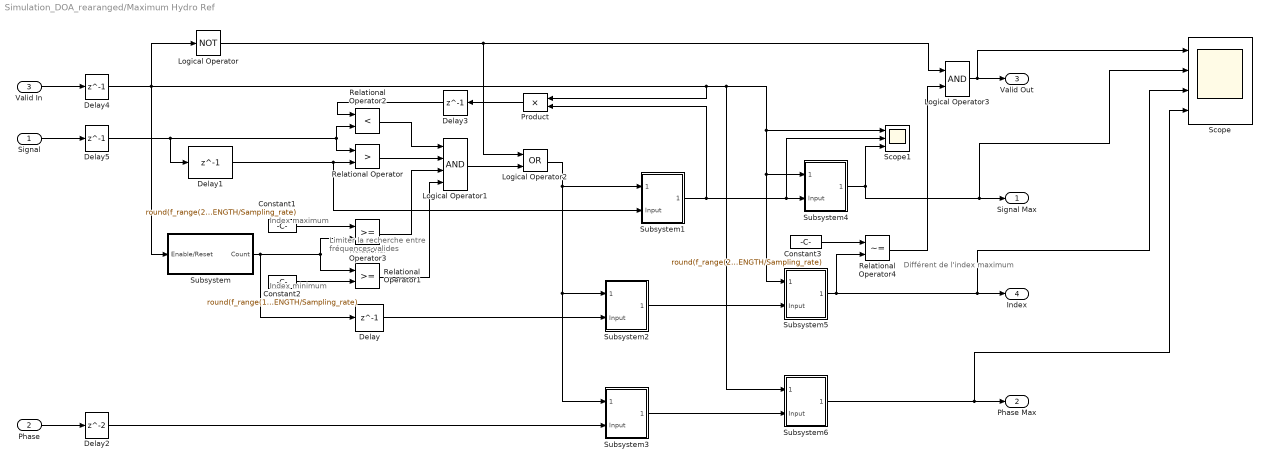
== system Simulation_DOA_rearanged/Maximum Hydro Ref ==
  note: Index minimum
  note: Index maximum
  note: Limiter la recherche
      | entre fréquences valides
  note: Différent de l'index
      | maximum
  Signal : Inport
  Phase : Inport  Port=2
  Valid In : Inport  Port=3
  Constant1 : Constant  Value=round(f_range(2)*FFT_LENGTH/Sampling_rate)  OutDataTypeStr=fixdt(0,6)  SampleTime=-1
  Constant2 : Constant  Value=round(f_range(1)*FFT_LENGTH/Sampling_rate)  OutDataTypeStr=fixdt(0,6)  SampleTime=-1
  Constant3 : Constant  Value=round(f_range(2)*FFT_LENGTH/Sampling_rate)  OutDataTypeStr=fixdt(0,6)  SampleTime=-1
  Delay : Delay  DelayLength=1  InitialCondition=0
  Delay{1,3..5} (4 alike) : Delay  DelayLength=1  InitialCondition=0  UseCircularBuffer=on
  Delay2 : Delay  InitialCondition=0  UseCircularBuffer=on
  Logical Operator : Logic  Operator=NOT  IconShape=distinctive  AllPortsSameDT=off  OutDataTypeStr=boolean
  Logical Operator1 : Logic  Inputs=4  AllPortsSameDT=off  OutDataTypeStr=boolean
  Logical Operator2 : Logic  Operator=OR  AllPortsSameDT=off  OutDataTypeStr=boolean
  Logical Operator3 : Logic  AllPortsSameDT=off  OutDataTypeStr=boolean
  Product : Product
  Relational Operator : RelationalOperator  Operator=>  OutDataTypeStr=boolean  RndMeth=Nearest
  Relational Operator1 : RelationalOperator  OutDataTypeStr=boolean  RndMeth=Nearest
  Relational Operator2 : RelationalOperator  Operator=<  OutDataTypeStr=boolean  RndMeth=Nearest
  Relational Operator3 : RelationalOperator  OutDataTypeStr=boolean  RndMeth=Nearest
  Relational Operator4 : RelationalOperator  Operator=~=  OutDataTypeStr=boolean  RndMeth=Nearest
  Scope : Scope  NumInputPorts=4
  Scope1 : Scope  NumInputPorts=3
  Subsystem : Subsystem
  Subsystem1 : Subsystem  TreatAsAtomicUnit=on
  Subsystem2 : Subsystem  TreatAsAtomicUnit=on
  Subsystem3 : Subsystem  TreatAsAtomicUnit=on
  Subsystem4 : Subsystem  TreatAsAtomicUnit=on
  Subsystem5 : Subsystem  TreatAsAtomicUnit=on
  Subsystem6 : Subsystem  TreatAsAtomicUnit=on
  Signal Max : Outport  VectorParamsAs1DForOutWhenUnconnected=off
  Phase Max : Outport  Port=2  VectorParamsAs1DForOutWhenUnconnected=off
  Valid Out : Outport  Port=3  VectorParamsAs1DForOutWhenUnconnected=off
  Index : Outport  Port=4  VectorParamsAs1DForOutWhenUnconnected=off
  wires:
  Subsystem1/1(" ") -> Product/2, Subsystem4/2(Input), Scope1/2
  Signal/1 -> Delay5/1
  Subsystem2/1(" ") -> Subsystem5/2(Input)
  Valid In/1 -> Delay4/1
  Delay1/1 -> Subsystem1/2(Input), Relational Operator/2
  Subsystem4/1(" ") -> Scope/2, Signal Max/1, Scope1/3
  Constant2/1 -> Relational Operator1/2
  Subsystem3/1(" ") -> Subsystem6/2(Input)
  Phase/1 -> Delay2/1
  Subsystem6/1(" ") -> Phase Max/1, Scope/4
  Subsystem/1(Count) -> Delay/1, Relational Operator1/1, Relational Operator3/2
  Relational Operator2/1 -> Logical Operator1/1
  Relational Operator/1 -> Logical Operator1/2
  Delay3/1 -> Relational Operator2/1
  Product/1 -> Delay3/1
  Delay4/1 -> Logical Operator/1, Subsystem6/1(Trigger), Subsystem5/1(Trigger), Subsystem4/1(Trigger), Scope1/1, Product/1, Subsystem/1(Enable/Reset)
  Delay5/1 -> Relational Operator2/2, Relational Operator/1, Delay1/1
  Delay2/1 -> Subsystem3/2(Input)
  Constant1/1 -> Relational Operator3/1
  Relational Operator1/1 -> Logical Operator1/4
  Logical Operator/1 -> Logical Operator2/1, Logical Operator3/1
  Logical Operator3/1 -> Scope/1, Valid Out/1
  Relational Operator3/1 -> Logical Operator1/3
  Relational Operator4/1 -> Logical Operator3/2
  Constant3/1 -> Relational Operator4/1
  Logical Operator1/1 -> Logical Operator2/2
  Logical Operator2/1 -> Subsystem1/1(Trigger), Subsystem3/1(Trigger), Subsystem2/1(Trigger)
  Delay/1 -> Subsystem2/2(Input)
  Subsystem5/1(" ") -> Index/1, Scope/3, Relational Operator4/2

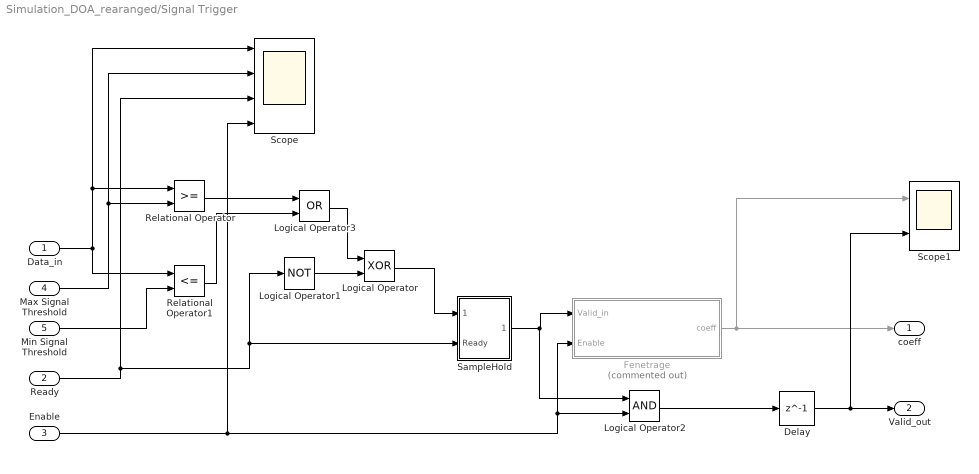
== system Simulation_DOA_rearanged/Signal Trigger ==
  Data_in : Inport
  Ready : Inport  Port=2  OutDataTypeStr=boolean
  Enable : Inport  Port=3  OutDataTypeStr=boolean
  Max Signal Threshold : Inport  Port=4
  Min Signal Threshold : Inport  Port=5
  Delay : Delay  DelayLength=1
  Fenetrage : Subsystem  Commented=on
  Logical Operator : Logic  Operator=XOR  AllPortsSameDT=off  OutDataTypeStr=boolean
  Logical Operator1 : Logic  Operator=NOT  IconShape=distinctive  AllPortsSameDT=off  OutDataTypeStr=boolean
  Logical Operator2 : Logic  AllPortsSameDT=off  OutDataTypeStr=boolean
  Logical Operator3 : Logic  Operator=OR  AllPortsSameDT=off  OutDataTypeStr=boolean
  Relational Operator : RelationalOperator  OutDataTypeStr=boolean  RndMeth=Nearest
  Relational Operator1 : RelationalOperator  Operator=<=  OutDataTypeStr=boolean  RndMeth=Nearest
  SampleHold : Subsystem  TreatAsAtomicUnit=on
  Scope : Scope  NumInputPorts=4
  Scope1 : Scope  NumInputPorts=2
  coeff : Outport
  Valid_out : Outport  Port=2
  wires:
  Data_in/1 -> Scope/1, Relational Operator/1, Relational Operator1/1
  Fenetrage/1(coeff) -> Scope1/1, coeff/1
  Logical Operator/1 -> SampleHold/1(Trigger)
  SampleHold/1(" ") -> Logical Operator2/1, Fenetrage/1(Valid_in)
  Logical Operator1/1 -> Logical Operator/2
  Enable/1 -> Scope/4, Logical Operator2/2, Fenetrage/2(Enable)
  Ready/1 -> Scope/3, Logical Operator1/1, SampleHold/2(Ready)
  Max Signal Threshold/1 -> Scope/2, Relational Operator/2
  Delay/1 -> Scope1/2, Valid_out/1
  Logical Operator2/1 -> Delay/1
  Relational Operator/1 -> Logical Operator3/1
  Logical Operator3/1 -> Logical Operator/1
  Min Signal Threshold/1 -> Relational Operator1/2
  Relational Operator1/1 -> Logical Operator3/2

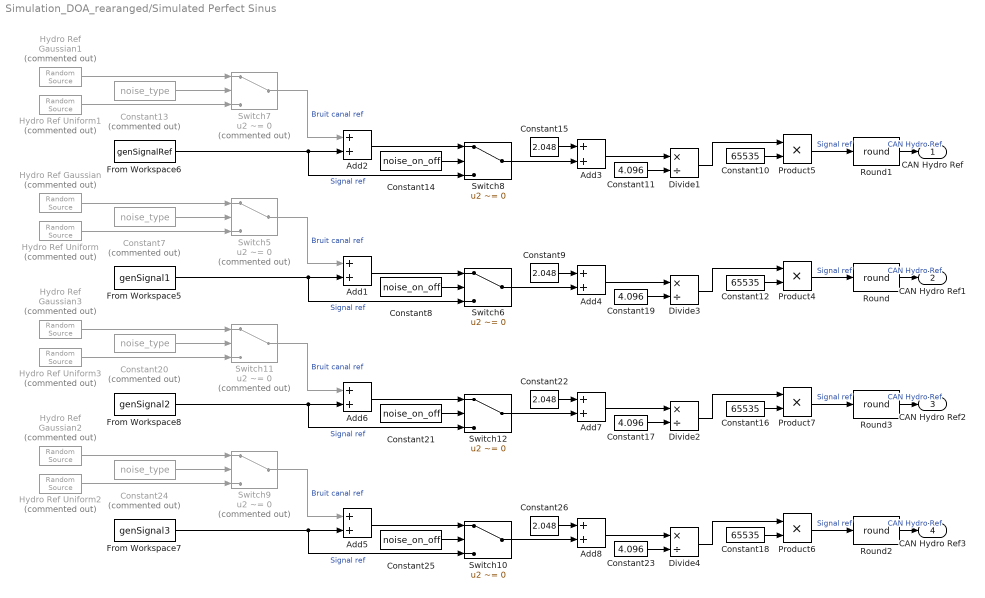
== system Simulation_DOA_rearanged/Simulated Perfect Sinus ==
  Add{1..8} (8 alike) : Sum
  Constant{10,12,16,18} (4 alike) : Constant  Value=65535  SampleTime=-1
  Constant{11,17,19,23} (4 alike) : Constant  Value=4.096  SampleTime=-1
  Constant{7,13,20,24} (4 alike) : Constant  Commented=on  Value=noise_type  VectorParams1D=off  SampleTime=-1
  Constant{8,14,21,25} (4 alike) : Constant  Value=noise_on_off  VectorParams1D=off  SampleTime=-1
  Constant{9,15,22,26} (4 alike) : Constant  Value=2.048  VectorParams1D=off  SampleTime=-1
  Divide{1..4} (4 alike) : Product  Inputs=*/
  From Workspace5 : FromWorkspace  VariableName=genSignal1  SampleTime=timePerSample  Interpolate=off  OutputAfterFinalValue=Setting to zero
  From Workspace6 : FromWorkspace  VariableName=genSignalRef  SampleTime=timePerSample  Interpolate=off  OutputAfterFinalValue=Setting to zero
  From Workspace7 : FromWorkspace  VariableName=genSignal3  SampleTime=timePerSample  Interpolate=off  OutputAfterFinalValue=Setting to zero
  From Workspace8 : FromWorkspace  VariableName=genSignal2  SampleTime=timePerSample  Interpolate=off  OutputAfterFinalValue=Setting to zero
  Hydro Ref Gaussian{,1..3} (4 alike) : dspsrcs4/Random Source  Commented=on  SrcType=Gaussian  NormMethod=Ziggurat  CltLength=12  MinVal=0  MaxVal=1  MeanVal=0  VarVal=variance  RepMode=Specify seed  rawSeed=randSeed1  IsInherit=off  SampMode=Discrete  SampTime=-1  SampFrame=1  DataType=Double  OutComplex=Real  OutputFrames=off
  Hydro Ref Uniform{,1..3} (4 alike) : dspsrcs4/Random Source  Commented=on  SrcType=Uniform  NormMethod=Ziggurat  CltLength=12  MinVal=-0.9  MaxVal=0.9  MeanVal=0  VarVal=1  RepMode=Specify seed  rawSeed=3409859  IsInherit=off  SampMode=Discrete  SampTime=-1  SampFrame=1  DataType=Double  OutComplex=Real  OutputFrames=off
  Product{4..7} (4 alike) : Product
  Round{,1..3} (4 alike) : Rounding  Operator=round
  Switch{6,8,10,12} (4 alike) : Switch  Criteria=u2 ~= 0
  Switch{5,7,9,11} (4 alike) : Switch  Commented=on  Criteria=u2 ~= 0
  CAN Hydro Ref : Outport
  CAN Hydro Ref1 : Outport  Port=2
  CAN Hydro Ref2 : Outport  Port=3
  CAN Hydro Ref3 : Outport  Port=4
  wires:
  Divide3/1 -> Product4/1
  Constant9/1 -> Add4/1
  Constant11/1 -> Divide1/2
  From Workspace7/1 -> Switch10/3, Add5/2  "Signal ref"
  Constant19/1 -> Divide3/2
  Hydro Ref Gaussian/1 -> Switch5/1
  Add2/1 -> Switch8/1
  Constant8/1 -> Switch6/2
  Add5/1 -> Switch10/1
  From Workspace5/1 -> Switch6/3, Add1/2  "Signal ref"
  Add3/1 -> Divide1/1
  Switch7/1 -> Add2/1  "Bruit canal ref"
  From Workspace6/1 -> Switch8/3, Add2/2  "Signal ref"
  Constant21/1 -> Switch12/2
  Constant7/1 -> Switch5/2
  Switch6/1 -> Add4/2
  Round3/1 -> CAN Hydro Ref2/1  "CAN Hydro Ref"
  Constant23/1 -> Divide4/2
  Constant17/1 -> Divide2/2
  Constant12/1 -> Product4/2
  Hydro Ref Gaussian3/1 -> Switch11/1
  Product4/1 -> Round/1  "Signal ref"
  Constant24/1 -> Switch9/2
  Switch9/1 -> Add5/1  "Bruit canal ref"
  Add4/1 -> Divide3/1
  Divide2/1 -> Product7/1
  Round2/1 -> CAN Hydro Ref3/1  "CAN Hydro Ref"
  Hydro Ref Uniform/1 -> Switch5/3
  Constant14/1 -> Switch8/2
  Switch5/1 -> Add1/1  "Bruit canal ref"
  Add8/1 -> Divide4/1
  Product7/1 -> Round3/1  "Signal ref"
  Constant10/1 -> Product5/2
  Constant16/1 -> Product7/2
  Hydro Ref Uniform3/1 -> Switch11/3
  Add1/1 -> Switch6/1
  Constant13/1 -> Switch7/2
  Constant15/1 -> Add3/1
  Hydro Ref Gaussian1/1 -> Switch7/1
  Switch8/1 -> Add3/2
  Divide1/1 -> Product5/1
  Product6/1 -> Round2/1  "Signal ref"
  Round1/1 -> CAN Hydro Ref/1  "CAN Hydro Ref"
  Constant18/1 -> Product6/2
  Product5/1 -> Round1/1  "Signal ref"
  Constant20/1 -> Switch11/2
  Switch11/1 -> Add6/1  "Bruit canal ref"
  From Workspace8/1 -> Switch12/3, Add6/2  "Signal ref"
  Hydro Ref Uniform1/1 -> Switch7/3
  Add6/1 -> Switch12/1
  Switch12/1 -> Add7/2
  Constant22/1 -> Add7/1
  Hydro Ref Uniform2/1 -> Switch9/3
  Divide4/1 -> Product6/1
  Constant26/1 -> Add8/1
  Switch10/1 -> Add8/2
  Hydro Ref Gaussian2/1 -> Switch9/1
  Add7/1 -> Divide2/1
  Round/1 -> CAN Hydro Ref1/1  "CAN Hydro Ref"
  Constant25/1 -> Switch10/2

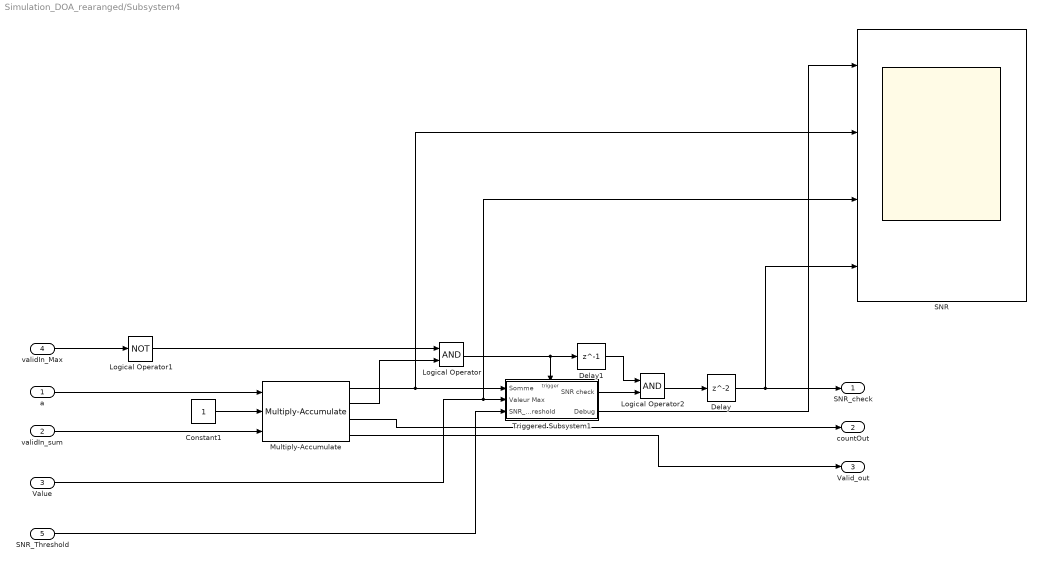
== system Simulation_DOA_rearanged/Subsystem4 ==
  a : Inport
  validIn_sum : Inport  Port=2
  " Value" : Inport  Port=3
  validIn_Max : Inport  Port=4
  SNR_Threshold : Inport  Port=5
  Constant1 : Constant  OutDataTypeStr=fixdt(1,27,8)  SampleTime=-1
  Delay : Delay
  Delay1 : Delay  DelayLength=1
  Logical Operator : Logic  AllPortsSameDT=off  OutDataTypeStr=boolean
  Logical Operator1 : Logic  Operator=NOT  AllPortsSameDT=off  OutDataTypeStr=boolean
  Logical Operator2 : Logic  AllPortsSameDT=off  OutDataTypeStr=boolean
  Multiply-Accumulate : hdlsllib/HDL Operations/Multiply-Accumulate  opMode=Streaming - using Number of Samples  initValueSetting=Dialog  initValue=0  initValueSetting2=Dialog  initValue2=0  initValueSetting3=Dialog  initValue3=0  num_samples=256  RndMeth2=Floor  RndMeth3=Floor  datatype2=Inherit: Inherit via back propagation  datatype3=fixdt(1,27,8)  validOut=on  endInandOut=on  startOut=on  countOut=on  dim=-1  DoSatur=off  parallel=off
      settings: SourceProductBaseCode=SL
  SNR : Scope  NumInputPorts=4
  Triggered Subsystem1 : Subsystem  TreatAsAtomicUnit=on
  SNR_check : Outport
  countOut : Outport  Port=2
  Valid_out : Outport  Port=3
  wires:
  validIn_sum/1 -> Multiply-Accumulate/3
  Constant1/1 -> Multiply-Accumulate/2
  Multiply-Accumulate/1 -> Triggered Subsystem1/1(Somme), SNR/2
  " Value"/1 -> Triggered Subsystem1/2(" Valeur Max"), SNR/3
  Multiply-Accumulate/3 -> countOut/1
  validIn_Max/1 -> Logical Operator1/1
  Logical Operator1/1 -> Logical Operator/1
  Multiply-Accumulate/2 -> Logical Operator/2
  Multiply-Accumulate/4 -> Valid_out/1
  a/1 -> Multiply-Accumulate/1
  Logical Operator/1 -> Delay1/1, Triggered Subsystem1/Trigger
  Delay/1 -> SNR/4, SNR_check/1
  Triggered Subsystem1/2(Debug) -> SNR/1
  SNR_Threshold/1 -> Triggered Subsystem1/3(SNR_Threshold)
  Triggered Subsystem1/1(SNR check) -> Logical Operator2/2
  Logical Operator2/1 -> Delay/1
  Delay1/1 -> Logical Operator2/1

== system Simulation_DOA_rearanged/Maximum Hydro 1/Subsystem ==
  Enable/Reset : Inport
  Add : Sum
  Data Type Conversion1 : DataTypeConversion  OutDataTypeStr=uint16  RndMeth=Nearest
  Delay : Delay  DelayLength=1  InitialCondition=0  UseCircularBuffer=on
  Product2 : Product
  Count : Outport  VectorParamsAs1DForOutWhenUnconnected=off
  wires:
  Enable/Reset/1 -> Add/1, Product2/1
  Add/1 -> Product2/2
  Delay/1 -> Count/1, Data Type Conversion1/1
  Product2/1 -> Delay/1
  Data Type Conversion1/1 -> Add/2

== system Simulation_DOA_rearanged/Maximum Hydro 1/Subsystem1 ==
  Trigger : Inport
  Input : Inport  Port=2
  Sample and Hold : dspsigops/Sample and Hold  trig=Falling edge  initCond=0  latchinput=off
  " " : Outport
  wires:
  Input/1 -> Sample and Hold/1
  Trigger/1 -> Sample and Hold/Trigger
  Sample and Hold/1 -> " "/1

== system Simulation_DOA_rearanged/Maximum Hydro 1/Subsystem2 ==
  Trigger : Inport
  Input : Inport  Port=2
  Sample and Hold : dspsigops/Sample and Hold  trig=Falling edge  initCond=0  latchinput=off
  " " : Outport
  wires:
  Input/1 -> Sample and Hold/1
  Trigger/1 -> Sample and Hold/Trigger
  Sample and Hold/1 -> " "/1

== system Simulation_DOA_rearanged/Maximum Hydro 1/Subsystem3 ==
  Trigger : Inport
  Input : Inport  Port=2
  Sample and Hold : dspsigops/Sample and Hold  trig=Falling edge  initCond=0  latchinput=off
  " " : Outport
  wires:
  Input/1 -> Sample and Hold/1
  Trigger/1 -> Sample and Hold/Trigger
  Sample and Hold/1 -> " "/1

== system Simulation_DOA_rearanged/Maximum Hydro 1/Subsystem4 ==
  Trigger : Inport
  Input : Inport  Port=2
  Sample and Hold : dspsigops/Sample and Hold  trig=Falling edge  initCond=0  latchinput=off
  " " : Outport
  wires:
  Input/1 -> Sample and Hold/1
  Trigger/1 -> Sample and Hold/Trigger
  Sample and Hold/1 -> " "/1

== system Simulation_DOA_rearanged/Maximum Hydro 1/Subsystem5 ==
  Trigger : Inport
  Input : Inport  Port=2
  Sample and Hold : dspsigops/Sample and Hold  trig=Falling edge  initCond=0  latchinput=off
  " " : Outport
  wires:
  Input/1 -> Sample and Hold/1
  Trigger/1 -> Sample and Hold/Trigger
  Sample and Hold/1 -> " "/1

== system Simulation_DOA_rearanged/Maximum Hydro 1/Subsystem6 ==
  Trigger : Inport
  Input : Inport  Port=2
  Sample and Hold : dspsigops/Sample and Hold  trig=Falling edge  initCond=0  latchinput=off
  " " : Outport
  wires:
  Input/1 -> Sample and Hold/1
  Trigger/1 -> Sample and Hold/Trigger
  Sample and Hold/1 -> " "/1

== system Simulation_DOA_rearanged/Maximum Hydro 2/Subsystem ==
  Enable/Reset : Inport
  Add : Sum
  Data Type Conversion1 : DataTypeConversion  OutDataTypeStr=uint16  RndMeth=Nearest
  Delay : Delay  DelayLength=1  InitialCondition=0  UseCircularBuffer=on
  Product2 : Product
  Count : Outport  VectorParamsAs1DForOutWhenUnconnected=off
  wires:
  Enable/Reset/1 -> Add/1, Product2/1
  Add/1 -> Product2/2
  Delay/1 -> Count/1, Data Type Conversion1/1
  Product2/1 -> Delay/1
  Data Type Conversion1/1 -> Add/2

== system Simulation_DOA_rearanged/Maximum Hydro 2/Subsystem1 ==
  Trigger : Inport
  Input : Inport  Port=2
  Sample and Hold : dspsigops/Sample and Hold  trig=Falling edge  initCond=0  latchinput=off
  " " : Outport
  wires:
  Input/1 -> Sample and Hold/1
  Trigger/1 -> Sample and Hold/Trigger
  Sample and Hold/1 -> " "/1

== system Simulation_DOA_rearanged/Maximum Hydro 2/Subsystem2 ==
  Trigger : Inport
  Input : Inport  Port=2
  Sample and Hold : dspsigops/Sample and Hold  trig=Falling edge  initCond=0  latchinput=off
  " " : Outport
  wires:
  Input/1 -> Sample and Hold/1
  Trigger/1 -> Sample and Hold/Trigger
  Sample and Hold/1 -> " "/1

== system Simulation_DOA_rearanged/Maximum Hydro 2/Subsystem3 ==
  Trigger : Inport
  Input : Inport  Port=2
  Sample and Hold : dspsigops/Sample and Hold  trig=Falling edge  initCond=0  latchinput=off
  " " : Outport
  wires:
  Input/1 -> Sample and Hold/1
  Trigger/1 -> Sample and Hold/Trigger
  Sample and Hold/1 -> " "/1

== system Simulation_DOA_rearanged/Maximum Hydro 2/Subsystem4 ==
  Trigger : Inport
  Input : Inport  Port=2
  Sample and Hold : dspsigops/Sample and Hold  trig=Falling edge  initCond=0  latchinput=off
  " " : Outport
  wires:
  Input/1 -> Sample and Hold/1
  Trigger/1 -> Sample and Hold/Trigger
  Sample and Hold/1 -> " "/1

== system Simulation_DOA_rearanged/Maximum Hydro 2/Subsystem5 ==
  Trigger : Inport
  Input : Inport  Port=2
  Sample and Hold : dspsigops/Sample and Hold  trig=Falling edge  initCond=0  latchinput=off
  " " : Outport
  wires:
  Input/1 -> Sample and Hold/1
  Trigger/1 -> Sample and Hold/Trigger
  Sample and Hold/1 -> " "/1

== system Simulation_DOA_rearanged/Maximum Hydro 2/Subsystem6 ==
  Trigger : Inport
  Input : Inport  Port=2
  Sample and Hold : dspsigops/Sample and Hold  trig=Falling edge  initCond=0  latchinput=off
  " " : Outport
  wires:
  Input/1 -> Sample and Hold/1
  Trigger/1 -> Sample and Hold/Trigger
  Sample and Hold/1 -> " "/1
